simulink model "final_fuzzy_modified_fullfuzzy"  (Simulink 7.4)
settings: Solver=ode23tb  StartTime=0.0  StopTime=0.5  MaxStep=1e-5  RelTol=1e-4
undefined symbols (not defined in the file): NEWFLC1
libraries: powerlib x25, powerlib_extras x3, fuzwiz x2, powerlib_models x1, fuzblock x1
(part 2 of 2)

== system final_fuzzy_modified_fullfuzzy/controller/Subsystem1/vector selector_0/compare and signal3 ==
  In1 : Inport
  In2 : Inport  Port=2
  logic_in : Inport  Port=3
  " 2" : Logic  AllPortsSameDT=off  OutDataTypeMode=boolean  OutDataTypeStr=boolean
  Clock1 : Clock
      settings: Decimation=10
  Relational Operator3 : RelationalOperator  LogicOutDataTypeMode=boolean  OutDataTypeStr=boolean
  Sum1 : Sum  Inputs=++|  OutDataType=sfix(16)  OutScaling=2^0
  logic_out : Outport
  sum : Outport  Port=2
  wires:
  logic_in/1 -> " 2"/2
  " 2"/1 -> logic_out/1
  In2/1 -> Sum1/2
  In1/1 -> Sum1/1
  Relational Operator3/1 -> " 2"/1
  Clock1/1 -> Relational Operator3/2
  Sum1/1 -> sum/1, Relational Operator3/1

== system final_fuzzy_modified_fullfuzzy/controller/Subsystem1/vector selector_0/compare and signal4 ==
  In1 : Inport
  In2 : Inport  Port=2
  logic_in : Inport  Port=3
  " 2" : Logic  AllPortsSameDT=off  OutDataTypeMode=boolean  OutDataTypeStr=boolean
  Clock1 : Clock
      settings: Decimation=10
  Relational Operator3 : RelationalOperator  LogicOutDataTypeMode=boolean  OutDataTypeStr=boolean
  Sum1 : Sum  Inputs=++|  OutDataType=sfix(16)  OutScaling=2^0
  logic_out : Outport
  sum : Outport  Port=2
  wires:
  Sum1/1 -> Relational Operator3/1, sum/1
  Clock1/1 -> Relational Operator3/2
  Relational Operator3/1 -> " 2"/1
  In1/1 -> Sum1/1
  In2/1 -> Sum1/2
  " 2"/1 -> logic_out/1
  logic_in/1 -> " 2"/2

== system final_fuzzy_modified_fullfuzzy/controller/Subsystem1/vector selector_0/compare and signal5 ==
  In1 : Inport
  In2 : Inport  Port=2
  logic_in : Inport  Port=3
  " 2" : Logic  AllPortsSameDT=off  OutDataTypeMode=boolean  OutDataTypeStr=boolean
  Clock1 : Clock
      settings: Decimation=10
  Relational Operator3 : RelationalOperator  LogicOutDataTypeMode=boolean  OutDataTypeStr=boolean
  Sum1 : Sum  Inputs=++|  OutDataType=sfix(16)  OutScaling=2^0
  logic_out : Outport
  sum : Outport  Port=2
  wires:
  Sum1/1 -> Relational Operator3/1, sum/1
  Clock1/1 -> Relational Operator3/2
  Relational Operator3/1 -> " 2"/1
  In1/1 -> Sum1/1
  In2/1 -> Sum1/2
  " 2"/1 -> logic_out/1
  logic_in/1 -> " 2"/2

== system final_fuzzy_modified_fullfuzzy/controller/Subsystem1/vector selector_1/compare and signal ==
  In1 : Inport
  In2 : Inport  Port=2
  logic_in : Inport  Port=3
  " 2" : Logic  AllPortsSameDT=off  OutDataTypeMode=boolean  OutDataTypeStr=boolean
  Clock1 : Clock
      settings: Decimation=10
  Relational Operator3 : RelationalOperator  LogicOutDataTypeMode=boolean  OutDataTypeStr=boolean
  Sum1 : Sum  Inputs=++|  OutDataType=sfix(16)  OutScaling=2^0
  logic_out : Outport
  sum : Outport  Port=2
  wires:
  logic_in/1 -> " 2"/2
  " 2"/1 -> logic_out/1
  In2/1 -> Sum1/2
  In1/1 -> Sum1/1
  Relational Operator3/1 -> " 2"/1
  Clock1/1 -> Relational Operator3/2
  Sum1/1 -> sum/1, Relational Operator3/1

== system final_fuzzy_modified_fullfuzzy/controller/Subsystem1/vector selector_1/compare and signal1 ==
  In1 : Inport
  In2 : Inport  Port=2
  logic_in : Inport  Port=3
  " 2" : Logic  AllPortsSameDT=off  OutDataTypeMode=boolean  OutDataTypeStr=boolean
  Clock1 : Clock
      settings: Decimation=10
  Relational Operator3 : RelationalOperator  LogicOutDataTypeMode=boolean  OutDataTypeStr=boolean
  Sum1 : Sum  Inputs=++|  OutDataType=sfix(16)  OutScaling=2^0
  logic_out : Outport
  sum : Outport  Port=2
  wires:
  Sum1/1 -> Relational Operator3/1, sum/1
  Clock1/1 -> Relational Operator3/2
  Relational Operator3/1 -> " 2"/1
  In1/1 -> Sum1/1
  In2/1 -> Sum1/2
  " 2"/1 -> logic_out/1
  logic_in/1 -> " 2"/2

== system final_fuzzy_modified_fullfuzzy/controller/Subsystem1/vector selector_1/compare and signal2 ==
  In1 : Inport
  In2 : Inport  Port=2
  logic_in : Inport  Port=3
  " 2" : Logic  AllPortsSameDT=off  OutDataTypeMode=boolean  OutDataTypeStr=boolean
  Clock1 : Clock
      settings: Decimation=10
  Relational Operator3 : RelationalOperator  LogicOutDataTypeMode=boolean  OutDataTypeStr=boolean
  Sum1 : Sum  Inputs=++|  OutDataType=sfix(16)  OutScaling=2^0
  logic_out : Outport
  sum : Outport  Port=2
  wires:
  logic_in/1 -> " 2"/2
  " 2"/1 -> logic_out/1
  In2/1 -> Sum1/2
  In1/1 -> Sum1/1
  Relational Operator3/1 -> " 2"/1
  Clock1/1 -> Relational Operator3/2
  Sum1/1 -> sum/1, Relational Operator3/1

== system final_fuzzy_modified_fullfuzzy/controller/Subsystem1/vector selector_1/compare and signal3 ==
  In1 : Inport
  In2 : Inport  Port=2
  logic_in : Inport  Port=3
  " 2" : Logic  AllPortsSameDT=off  OutDataTypeMode=boolean  OutDataTypeStr=boolean
  Clock1 : Clock
      settings: Decimation=10
  Relational Operator3 : RelationalOperator  LogicOutDataTypeMode=boolean  OutDataTypeStr=boolean
  Sum1 : Sum  Inputs=++|  OutDataType=sfix(16)  OutScaling=2^0
  logic_out : Outport
  sum : Outport  Port=2
  wires:
  Sum1/1 -> Relational Operator3/1, sum/1
  Clock1/1 -> Relational Operator3/2
  Relational Operator3/1 -> " 2"/1
  In1/1 -> Sum1/1
  In2/1 -> Sum1/2
  " 2"/1 -> logic_out/1
  logic_in/1 -> " 2"/2

== system final_fuzzy_modified_fullfuzzy/controller/Subsystem1/vector selector_1/compare and signal4 ==
  In1 : Inport
  In2 : Inport  Port=2
  logic_in : Inport  Port=3
  " 2" : Logic  AllPortsSameDT=off  OutDataTypeMode=boolean  OutDataTypeStr=boolean
  Clock1 : Clock
      settings: Decimation=10
  Relational Operator3 : RelationalOperator  LogicOutDataTypeMode=boolean  OutDataTypeStr=boolean
  Sum1 : Sum  Inputs=++|  OutDataType=sfix(16)  OutScaling=2^0
  logic_out : Outport
  sum : Outport  Port=2
  wires:
  logic_in/1 -> " 2"/2
  " 2"/1 -> logic_out/1
  In2/1 -> Sum1/2
  In1/1 -> Sum1/1
  Relational Operator3/1 -> " 2"/1
  Clock1/1 -> Relational Operator3/2
  Sum1/1 -> sum/1, Relational Operator3/1

== system final_fuzzy_modified_fullfuzzy/controller/Subsystem1/vector selector_1/compare and signal5 ==
  In1 : Inport
  In2 : Inport  Port=2
  logic_in : Inport  Port=3
  " 2" : Logic  AllPortsSameDT=off  OutDataTypeMode=boolean  OutDataTypeStr=boolean
  Clock1 : Clock
      settings: Decimation=10
  Relational Operator3 : RelationalOperator  LogicOutDataTypeMode=boolean  OutDataTypeStr=boolean
  Sum1 : Sum  Inputs=++|  OutDataType=sfix(16)  OutScaling=2^0
  logic_out : Outport
  sum : Outport  Port=2
  wires:
  logic_in/1 -> " 2"/2
  " 2"/1 -> logic_out/1
  In2/1 -> Sum1/2
  In1/1 -> Sum1/1
  Relational Operator3/1 -> " 2"/1
  Clock1/1 -> Relational Operator3/2
  Sum1/1 -> sum/1, Relational Operator3/1

== system final_fuzzy_modified_fullfuzzy/controller/Subsystem2/vector selector_0/compare and signal ==
  In1 : Inport
  In2 : Inport  Port=2
  logic_in : Inport  Port=3
  " 2" : Logic  AllPortsSameDT=off  OutDataTypeMode=boolean  OutDataTypeStr=boolean
  Clock1 : Clock
      settings: Decimation=10
  Relational Operator3 : RelationalOperator  LogicOutDataTypeMode=boolean  OutDataTypeStr=boolean
  Sum1 : Sum  Inputs=++|  OutDataType=sfix(16)  OutScaling=2^0
  logic_out : Outport
  sum : Outport  Port=2
  wires:
  logic_in/1 -> " 2"/2
  " 2"/1 -> logic_out/1
  In2/1 -> Sum1/2
  In1/1 -> Sum1/1
  Relational Operator3/1 -> " 2"/1
  Clock1/1 -> Relational Operator3/2
  Sum1/1 -> sum/1, Relational Operator3/1

== system final_fuzzy_modified_fullfuzzy/controller/Subsystem2/vector selector_0/compare and signal1 ==
  In1 : Inport
  In2 : Inport  Port=2
  logic_in : Inport  Port=3
  " 2" : Logic  AllPortsSameDT=off  OutDataTypeMode=boolean  OutDataTypeStr=boolean
  Clock1 : Clock
      settings: Decimation=10
  Relational Operator3 : RelationalOperator  LogicOutDataTypeMode=boolean  OutDataTypeStr=boolean
  Sum1 : Sum  Inputs=++|  OutDataType=sfix(16)  OutScaling=2^0
  logic_out : Outport
  sum : Outport  Port=2
  wires:
  Sum1/1 -> Relational Operator3/1, sum/1
  Clock1/1 -> Relational Operator3/2
  Relational Operator3/1 -> " 2"/1
  In1/1 -> Sum1/1
  In2/1 -> Sum1/2
  " 2"/1 -> logic_out/1
  logic_in/1 -> " 2"/2

== system final_fuzzy_modified_fullfuzzy/controller/Subsystem2/vector selector_0/compare and signal2 ==
  In1 : Inport
  In2 : Inport  Port=2
  logic_in : Inport  Port=3
  " 2" : Logic  AllPortsSameDT=off  OutDataTypeMode=boolean  OutDataTypeStr=boolean
  Clock1 : Clock
      settings: Decimation=10
  Relational Operator3 : RelationalOperator  LogicOutDataTypeMode=boolean  OutDataTypeStr=boolean
  Sum1 : Sum  Inputs=++|  OutDataType=sfix(16)  OutScaling=2^0
  logic_out : Outport
  sum : Outport  Port=2
  wires:
  logic_in/1 -> " 2"/2
  " 2"/1 -> logic_out/1
  In2/1 -> Sum1/2
  In1/1 -> Sum1/1
  Relational Operator3/1 -> " 2"/1
  Clock1/1 -> Relational Operator3/2
  Sum1/1 -> sum/1, Relational Operator3/1

== system final_fuzzy_modified_fullfuzzy/controller/Subsystem2/vector selector_0/compare and signal3 ==
  In1 : Inport
  In2 : Inport  Port=2
  logic_in : Inport  Port=3
  " 2" : Logic  AllPortsSameDT=off  OutDataTypeMode=boolean  OutDataTypeStr=boolean
  Clock1 : Clock
      settings: Decimation=10
  Relational Operator3 : RelationalOperator  LogicOutDataTypeMode=boolean  OutDataTypeStr=boolean
  Sum1 : Sum  Inputs=++|  OutDataType=sfix(16)  OutScaling=2^0
  logic_out : Outport
  sum : Outport  Port=2
  wires:
  Sum1/1 -> Relational Operator3/1, sum/1
  Clock1/1 -> Relational Operator3/2
  Relational Operator3/1 -> " 2"/1
  In1/1 -> Sum1/1
  In2/1 -> Sum1/2
  " 2"/1 -> logic_out/1
  logic_in/1 -> " 2"/2

== system final_fuzzy_modified_fullfuzzy/controller/Subsystem2/vector selector_0/compare and signal4 ==
  In1 : Inport
  In2 : Inport  Port=2
  logic_in : Inport  Port=3
  " 2" : Logic  AllPortsSameDT=off  OutDataTypeMode=boolean  OutDataTypeStr=boolean
  Clock1 : Clock
      settings: Decimation=10
  Relational Operator3 : RelationalOperator  LogicOutDataTypeMode=boolean  OutDataTypeStr=boolean
  Sum1 : Sum  Inputs=++|  OutDataType=sfix(16)  OutScaling=2^0
  logic_out : Outport
  sum : Outport  Port=2
  wires:
  logic_in/1 -> " 2"/2
  " 2"/1 -> logic_out/1
  In2/1 -> Sum1/2
  In1/1 -> Sum1/1
  Relational Operator3/1 -> " 2"/1
  Clock1/1 -> Relational Operator3/2
  Sum1/1 -> sum/1, Relational Operator3/1

== system final_fuzzy_modified_fullfuzzy/controller/Subsystem2/vector selector_0/compare and signal5 ==
  In1 : Inport
  In2 : Inport  Port=2
  logic_in : Inport  Port=3
  " 2" : Logic  AllPortsSameDT=off  OutDataTypeMode=boolean  OutDataTypeStr=boolean
  Clock1 : Clock
      settings: Decimation=10
  Relational Operator3 : RelationalOperator  LogicOutDataTypeMode=boolean  OutDataTypeStr=boolean
  Sum1 : Sum  Inputs=++|  OutDataType=sfix(16)  OutScaling=2^0
  logic_out : Outport
  sum : Outport  Port=2
  wires:
  logic_in/1 -> " 2"/2
  " 2"/1 -> logic_out/1
  In2/1 -> Sum1/2
  In1/1 -> Sum1/1
  Relational Operator3/1 -> " 2"/1
  Clock1/1 -> Relational Operator3/2
  Sum1/1 -> sum/1, Relational Operator3/1

== system final_fuzzy_modified_fullfuzzy/controller/Subsystem2/vector selector_1/compare and signal ==
  In1 : Inport
  In2 : Inport  Port=2
  logic_in : Inport  Port=3
  " 2" : Logic  AllPortsSameDT=off  OutDataTypeMode=boolean  OutDataTypeStr=boolean
  Clock1 : Clock
      settings: Decimation=10
  Relational Operator3 : RelationalOperator  LogicOutDataTypeMode=boolean  OutDataTypeStr=boolean
  Sum1 : Sum  Inputs=++|  OutDataType=sfix(16)  OutScaling=2^0
  logic_out : Outport
  sum : Outport  Port=2
  wires:
  Sum1/1 -> Relational Operator3/1, sum/1
  Clock1/1 -> Relational Operator3/2
  Relational Operator3/1 -> " 2"/1
  In1/1 -> Sum1/1
  In2/1 -> Sum1/2
  " 2"/1 -> logic_out/1
  logic_in/1 -> " 2"/2

== system final_fuzzy_modified_fullfuzzy/controller/Subsystem2/vector selector_1/compare and signal1 ==
  In1 : Inport
  In2 : Inport  Port=2
  logic_in : Inport  Port=3
  " 2" : Logic  AllPortsSameDT=off  OutDataTypeMode=boolean  OutDataTypeStr=boolean
  Clock1 : Clock
      settings: Decimation=10
  Relational Operator3 : RelationalOperator  LogicOutDataTypeMode=boolean  OutDataTypeStr=boolean
  Sum1 : Sum  Inputs=++|  OutDataType=sfix(16)  OutScaling=2^0
  logic_out : Outport
  sum : Outport  Port=2
  wires:
  logic_in/1 -> " 2"/2
  " 2"/1 -> logic_out/1
  In2/1 -> Sum1/2
  In1/1 -> Sum1/1
  Relational Operator3/1 -> " 2"/1
  Clock1/1 -> Relational Operator3/2
  Sum1/1 -> sum/1, Relational Operator3/1

== system final_fuzzy_modified_fullfuzzy/controller/Subsystem2/vector selector_1/compare and signal2 ==
  In1 : Inport
  In2 : Inport  Port=2
  logic_in : Inport  Port=3
  " 2" : Logic  AllPortsSameDT=off  OutDataTypeMode=boolean  OutDataTypeStr=boolean
  Clock1 : Clock
      settings: Decimation=10
  Relational Operator3 : RelationalOperator  LogicOutDataTypeMode=boolean  OutDataTypeStr=boolean
  Sum1 : Sum  Inputs=++|  OutDataType=sfix(16)  OutScaling=2^0
  logic_out : Outport
  sum : Outport  Port=2
  wires:
  Sum1/1 -> Relational Operator3/1, sum/1
  Clock1/1 -> Relational Operator3/2
  Relational Operator3/1 -> " 2"/1
  In1/1 -> Sum1/1
  In2/1 -> Sum1/2
  " 2"/1 -> logic_out/1
  logic_in/1 -> " 2"/2

== system final_fuzzy_modified_fullfuzzy/controller/Subsystem2/vector selector_1/compare and signal3 ==
  In1 : Inport
  In2 : Inport  Port=2
  logic_in : Inport  Port=3
  " 2" : Logic  AllPortsSameDT=off  OutDataTypeMode=boolean  OutDataTypeStr=boolean
  Clock1 : Clock
      settings: Decimation=10
  Relational Operator3 : RelationalOperator  LogicOutDataTypeMode=boolean  OutDataTypeStr=boolean
  Sum1 : Sum  Inputs=++|  OutDataType=sfix(16)  OutScaling=2^0
  logic_out : Outport
  sum : Outport  Port=2
  wires:
  logic_in/1 -> " 2"/2
  " 2"/1 -> logic_out/1
  In2/1 -> Sum1/2
  In1/1 -> Sum1/1
  Relational Operator3/1 -> " 2"/1
  Clock1/1 -> Relational Operator3/2
  Sum1/1 -> sum/1, Relational Operator3/1

== system final_fuzzy_modified_fullfuzzy/controller/Subsystem2/vector selector_1/compare and signal4 ==
  In1 : Inport
  In2 : Inport  Port=2
  logic_in : Inport  Port=3
  " 2" : Logic  AllPortsSameDT=off  OutDataTypeMode=boolean  OutDataTypeStr=boolean
  Clock1 : Clock
      settings: Decimation=10
  Relational Operator3 : RelationalOperator  LogicOutDataTypeMode=boolean  OutDataTypeStr=boolean
  Sum1 : Sum  Inputs=++|  OutDataType=sfix(16)  OutScaling=2^0
  logic_out : Outport
  sum : Outport  Port=2
  wires:
  Sum1/1 -> Relational Operator3/1, sum/1
  Clock1/1 -> Relational Operator3/2
  Relational Operator3/1 -> " 2"/1
  In1/1 -> Sum1/1
  In2/1 -> Sum1/2
  " 2"/1 -> logic_out/1
  logic_in/1 -> " 2"/2

== system final_fuzzy_modified_fullfuzzy/controller/Subsystem2/vector selector_1/compare and signal5 ==
  In1 : Inport
  In2 : Inport  Port=2
  logic_in : Inport  Port=3
  " 2" : Logic  AllPortsSameDT=off  OutDataTypeMode=boolean  OutDataTypeStr=boolean
  Clock1 : Clock
      settings: Decimation=10
  Relational Operator3 : RelationalOperator  LogicOutDataTypeMode=boolean  OutDataTypeStr=boolean
  Sum1 : Sum  Inputs=++|  OutDataType=sfix(16)  OutScaling=2^0
  logic_out : Outport
  sum : Outport  Port=2
  wires:
  Sum1/1 -> Relational Operator3/1, sum/1
  Clock1/1 -> Relational Operator3/2
  Relational Operator3/1 -> " 2"/1
  In1/1 -> Sum1/1
  In2/1 -> Sum1/2
  " 2"/1 -> logic_out/1
  logic_in/1 -> " 2"/2

== system final_fuzzy_modified_fullfuzzy/controller/Subsystem3/Fuzzy Logic  Controller/PI5 ==
  In1 : Inport  OutDataType=sfix(16)  OutScaling=2^0
  Gain2 : Gain  Gain=10  ParameterDataType=sfix(16)  ParameterScaling=2^0  OutDataType=sfix(16)  OutScaling=2^0
  Gain3 : Gain  Gain=500  ParameterDataType=sfix(16)  ParameterScaling=2^0  OutDataType=sfix(16)  OutScaling=2^0
  Integrator : Integrator  UpperSaturationLimit=1  LowerSaturationLimit=-1
  Sum7 : Sum  OutDataType=sfix(16)  OutScaling=2^0
  Out1 : Outport  OutDataType=sfix(16)  OutScaling=2^0
  wires:
  Gain3/1 -> Integrator/1
  Gain2/1 -> Sum7/1
  Integrator/1 -> Sum7/2
  In1/1 -> Gain2/1, Gain3/1
  Sum7/1 -> Out1/1

== system final_fuzzy_modified_fullfuzzy/controller/Subsystem4/Fuzzy Logic  Controller/PI2 ==
  In1 : Inport  OutDataType=sfix(16)  OutScaling=2^0
  Gain2 : Gain  Gain=1490  ParameterDataType=sfix(16)  ParameterScaling=2^0  OutDataType=sfix(16)  OutScaling=2^0
  Gain3 : Gain  Gain=1000  ParameterDataType=sfix(16)  ParameterScaling=2^0  OutDataType=sfix(16)  OutScaling=2^0
  Integrator : Integrator  UpperSaturationLimit=1  LowerSaturationLimit=-1
  Sum7 : Sum  OutDataType=sfix(16)  OutScaling=2^0
  Out1 : Outport  OutDataType=sfix(16)  OutScaling=2^0
  wires:
  Gain3/1 -> Integrator/1
  Gain2/1 -> Sum7/1
  Integrator/1 -> Sum7/2
  In1/1 -> Gain2/1, Gain3/1
  Sum7/1 -> Out1/1

== system final_fuzzy_modified_fullfuzzy/controller/Subsystem5/Fuzzy Logic  Controller/PI1 ==
  In1 : Inport  OutDataType=sfix(16)  OutScaling=2^0
  Gain2 : Gain  Gain=10  ParameterDataType=sfix(16)  ParameterScaling=2^0  OutDataType=sfix(16)  OutScaling=2^0
  Gain3 : Gain  Gain=1000  ParameterDataType=sfix(16)  ParameterScaling=2^0  OutDataType=sfix(16)  OutScaling=2^0
  Integrator : Integrator  LimitOutput=on  UpperSaturationLimit=1  LowerSaturationLimit=-1
  Sum7 : Sum  OutDataType=sfix(16)  OutScaling=2^0
  Out1 : Outport  OutDataType=sfix(16)  OutScaling=2^0
  wires:
  Sum7/1 -> Out1/1
  In1/1 -> Gain3/1, Gain2/1
  Integrator/1 -> Sum7/2
  Gain2/1 -> Sum7/1
  Gain3/1 -> Integrator/1
